simulink library "NLGCToolbox"  (R2017b)
settings: Solver=VariableStepAuto  StartTime=0.0  StopTime=10.0  RelTol=1e-3
undefined symbols (not defined in the file or in its folder): quadModel
libraries: simulink x8, NLGCToolbox x4
settings Model: Creator=hoang  LastModifiedBy=hoang

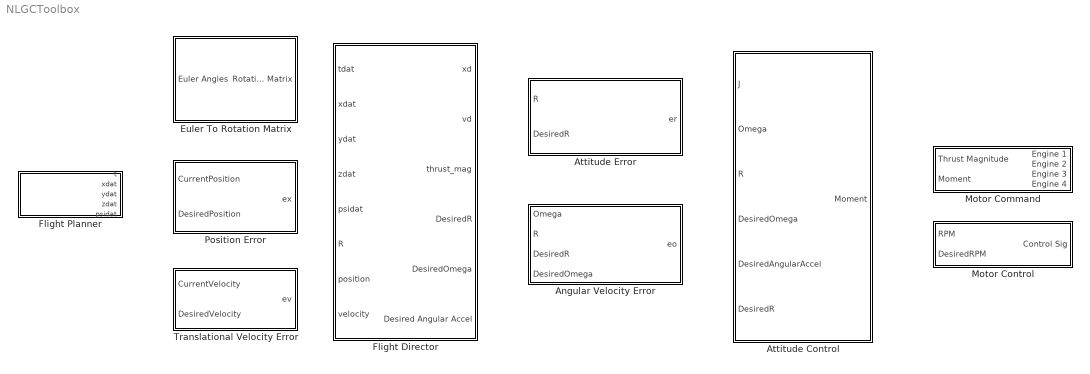
== system NLGCToolbox ==
  Angular Velocity Error : Subsystem
      settings: OpenFcn=set_param(gcbh,'LinkStatus','none');
  Attitude Control : Subsystem  mask{kr=12, ko=4}
      mask prompts: kr "Attitude error gain (Kr)"; ko "Angular velocity error gain (Ko)"
      mask init:
      | set_param(gcb, 'MaskSelfModifiable', 'on');
      settings: OpenFcn=set_param(gcbh,'LinkStatus','none');
  Attitude Error : Subsystem
      settings: OpenFcn=set_param(gcbh,'LinkStatus','none');
  Euler To Rotation Matrix : Subsystem
      settings: OpenFcn=set_param(gcbh,'LinkStatus','none');
  Flight Director : Subsystem  mask{Ts=0, kx=0, kv=0}
      mask prompts: Ts "Sampling Time (Ts)"; kx "Position Control Gain (kx)"; kv "Velocity Control Gain (kv)"
      settings: OpenFcn=set_param(gcbh,'LinkStatus','none');
  "Flight Planner " : Subsystem  mask{t=0, x=0, y=0, z=0, psi=0}
      mask prompts: t "Workspace Time Var"; x "Workspace x Var"; y "Workspace y Var"; z "Workspace z Var"; psi "Workspace psi Var"
      settings: OpenFcn=set_param(gcbh,'LinkStatus','none');
  Motor Command : Subsystem  mask{Ct=0, d=0, Cq=0}
      mask prompts: Ct "Force coefficient (Ct)"; d "Arm's length (d)"; Cq "Reaction torque coefficient (Cq)"
      settings: OpenFcn=set_param(gcbh,'LinkStatus','none');
  Motor Control : Subsystem  mask{k=0, Km=0, Ts=0, T=0, Rdt=0, Rdx=0, b=0}
      mask prompts: k "Velocity Gain (k)"; Km "Motor Amplification (Km)"; Ts "Sampling Time (Ts)"; T "Motor Time Constant (T)"; Rdt "Maximum Output Threshold (Rdt)"; Rdx "Maximum Derivative Threshold (Rdx)"; b "Throttle Bias"
      settings: OpenFcn=set_param(gcbh,'LinkStatus','none');
  Position Error : Subsystem
      settings: OpenFcn=set_param(gcbh,'LinkStatus','none');
  Translational Velocity Error : Subsystem
      settings: OpenFcn=set_param(gcbh,'LinkStatus','none');

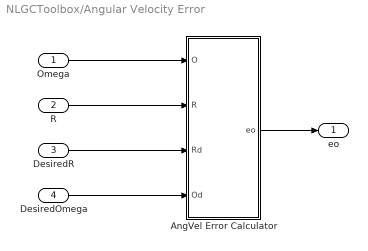
== system NLGCToolbox/Angular Velocity Error ==
  Omega : Inport
  R : Inport  Port=2
  DesiredR : Inport  Port=3
  DesiredOmega : Inport  Port=4
  AngVel Error Calculator : MATLAB Function  TreatAsAtomicUnit=on
  eo : Outport
  wires:
  Omega/1 -> AngVel Error Calculator/1(O)
  R/1 -> AngVel Error Calculator/2(R)
  DesiredR/1 -> AngVel Error Calculator/3(Rd)
  DesiredOmega/1 -> AngVel Error Calculator/4(Od)
  AngVel Error Calculator/1(eo) -> eo/1

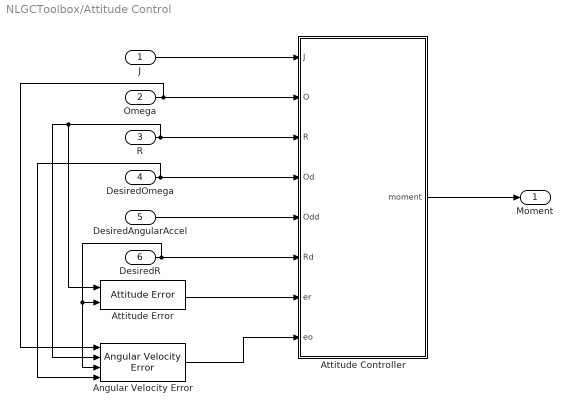
== system NLGCToolbox/Attitude Control ==
  J : Inport
  Omega : Inport  Port=2
  R : Inport  Port=3
  DesiredOmega : Inport  Port=4
  DesiredAngularAccel : Inport  Port=5
  DesiredR : Inport  Port=6
  Angular Velocity Error : NLGCToolbox/Angular Velocity Error
      settings: SourceProductName=Thinh - NLGC for Quadrotor
  Attitude Controller : MATLAB Function  TreatAsAtomicUnit=on
  Attitude Error : NLGCToolbox/Attitude Error
      settings: SourceProductName=Thinh - NLGC for Quadrotor
  Moment : Outport
  wires:
  Attitude Controller/1(moment) -> Moment/1
  DesiredR/1 -> Angular Velocity Error/3, Attitude Error/2, Attitude Controller/6(Rd)
  DesiredAngularAccel/1 -> Attitude Controller/5(Odd)
  DesiredOmega/1 -> Angular Velocity Error/4, Attitude Controller/4(Od)
  R/1 -> Attitude Error/1, Angular Velocity Error/2, Attitude Controller/3(R)
  Omega/1 -> Angular Velocity Error/1, Attitude Controller/2(O)
  J/1 -> Attitude Controller/1(J)
  Attitude Error/1 -> Attitude Controller/7(er)
  Angular Velocity Error/1 -> Attitude Controller/8(eo)

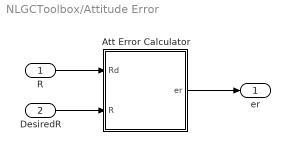
== system NLGCToolbox/Attitude Error ==
  R : Inport
  DesiredR : Inport  Port=2
  Att Error Calculator : MATLAB Function  TreatAsAtomicUnit=on
  er : Outport
  wires:
  Att Error Calculator/1(er) -> er/1
  R/1 -> Att Error Calculator/1(Rd)
  DesiredR/1 -> Att Error Calculator/2(R)

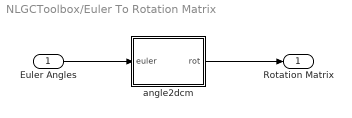
== system NLGCToolbox/Euler To Rotation Matrix ==
  Euler Angles : Inport
  angle2dcm : MATLAB Function  TreatAsAtomicUnit=on
  Rotation Matrix : Outport
  wires:
  Euler Angles/1 -> angle2dcm/1(euler)
  angle2dcm/1(rot) -> Rotation Matrix/1

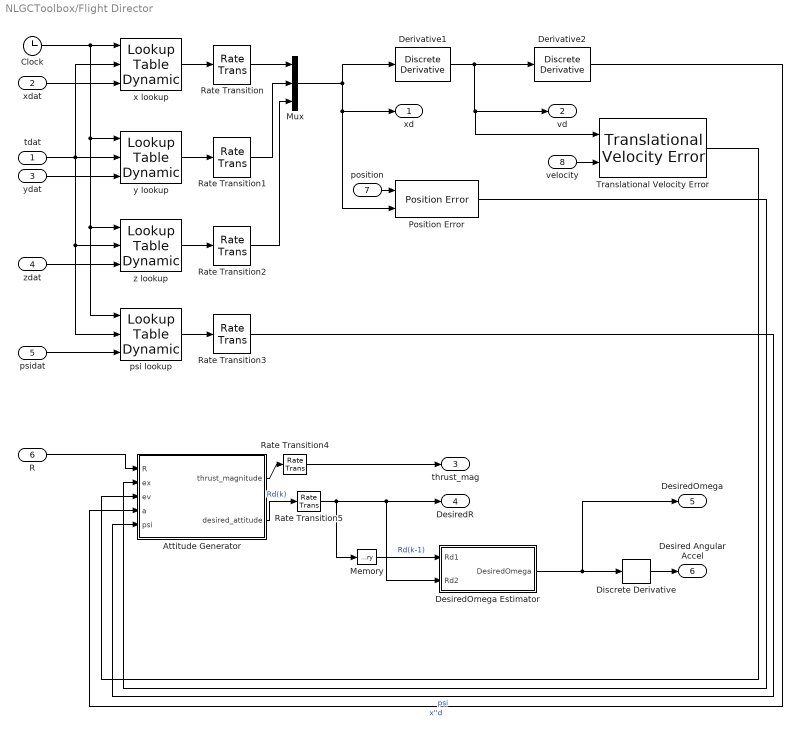
== system NLGCToolbox/Flight Director ==
  tdat : Inport
  xdat : Inport  Port=2
  ydat : Inport  Port=3
  zdat : Inport  Port=4
  psidat : Inport  Port=5
  R : Inport  Port=6
  position : Inport  Port=7
  velocity : Inport  Port=8
  Attitude Generator : MATLAB Function  TreatAsAtomicUnit=on
  Clock : Clock
  Derivative1 : simulink/Discrete/Discrete Derivative  gainval=1.0  ICPrevScaledInput=0.0  OutMin=[]  OutMax=[]  OutDataType=fixdt(1, 16)  OutScaling=2^-10  DoSatur=off
  Derivative2 : simulink/Discrete/Discrete Derivative  gainval=1.0  ICPrevScaledInput=0.0  OutMin=[]  OutMax=[]  OutDataType=fixdt(1, 16)  OutScaling=2^-10  DoSatur=off
  DesiredOmega Estimator : MATLAB Function  TreatAsAtomicUnit=on
  Discrete Derivative : simulink/Discrete/Discrete Derivative  gainval=1.0  ICPrevScaledInput=0.0  OutMin=[]  OutMax=[]  OutDataType=fixdt(1, 16)  OutScaling=2^-10  DoSatur=off
  Memory : Memory
  Mux : Mux  Inputs=3
  Position Error : NLGCToolbox/Position Error
      settings: SourceProductName=Thinh - NLGC for Quadrotor
  Rate Transition{,1..5} (6 alike) : RateTransition  OutPortSampleTime=Ts
  Translational Velocity Error : NLGCToolbox/Translational Velocity Error
      settings: SourceProductName=Thinh - NLGC for Quadrotor
  psi lookup : simulink/Lookup Tables/Lookup Table Dynamic  LookUpMeth=Interpolation-Use End Values  OutDataType=fixdt('double')  OutScaling=[]  OutputDataTypeScalingMode=Specify via dialog  OutDataTypeStr=double  DoSatur=off
      settings: SourceProductName=Simulink
  x lookup : simulink/Lookup Tables/Lookup Table Dynamic  LookUpMeth=Interpolation-Use End Values  OutDataType=fixdt('double')  OutScaling=[]  OutputDataTypeScalingMode=Specify via dialog  OutDataTypeStr=double  DoSatur=off
      settings: SourceProductName=Simulink
  y lookup : simulink/Lookup Tables/Lookup Table Dynamic  LookUpMeth=Interpolation-Use End Values  OutDataType=fixdt('double')  OutScaling=[]  OutputDataTypeScalingMode=Specify via dialog  OutDataTypeStr=double  DoSatur=off
      settings: SourceProductName=Simulink
  z lookup : simulink/Lookup Tables/Lookup Table Dynamic  LookUpMeth=Interpolation-Use End Values  OutDataType=fixdt('double')  OutScaling=[]  OutputDataTypeScalingMode=Specify via dialog  OutDataTypeStr=double  DoSatur=off
      settings: SourceProductName=Simulink
  xd : Outport
  vd : Outport  Port=2
  thrust_mag : Outport  Port=3
  DesiredR : Outport  Port=4
  DesiredOmega : Outport  Port=5
  Desired Angular Accel : Outport  Port=6
  wires:
  tdat/1 -> psi lookup/2, z lookup/2, x lookup/2, y lookup/2
  Clock/1 -> psi lookup/1, z lookup/1, y lookup/1, x lookup/1
  xdat/1 -> x lookup/3
  ydat/1 -> y lookup/3
  zdat/1 -> z lookup/3
  x lookup/1 -> Rate Transition/1
  y lookup/1 -> Rate Transition1/1
  z lookup/1 -> Rate Transition2/1
  Rate Transition/1 -> Mux/1
  Rate Transition1/1 -> Mux/2
  Rate Transition2/1 -> Mux/3
  Derivative1/1 -> Translational Velocity Error/1, vd/1, Derivative2/1
  psi lookup/1 -> Rate Transition3/1
  Derivative2/1 -> Attitude Generator/4(a)  "x''d"
  Rate Transition3/1 -> Attitude Generator/5(psi)  "psi"
  Attitude Generator/1(thrust_magnitude) -> Rate Transition4/1
  Attitude Generator/2(desired_attitude) -> Rate Transition5/1  "Rd(k)"
  R/1 -> Attitude Generator/1(R)
  DesiredOmega Estimator/1(DesiredOmega) -> Discrete Derivative/1, DesiredOmega/1
  Discrete Derivative/1 -> Desired Angular Accel/1
  Rate Transition5/1 -> Memory/1, DesiredOmega Estimator/2(Rd2), DesiredR/1
  Rate Transition4/1 -> thrust_mag/1
  Memory/1 -> DesiredOmega Estimator/1(Rd1)  "Rd(k-1)"
  Mux/1 -> xd/1, Position Error/2, Derivative1/1
  position/1 -> Position Error/1
  Position Error/1 -> Attitude Generator/2(ex)
  velocity/1 -> Translational Velocity Error/2
  Translational Velocity Error/1 -> Attitude Generator/3(ev)
  psidat/1 -> psi lookup/3

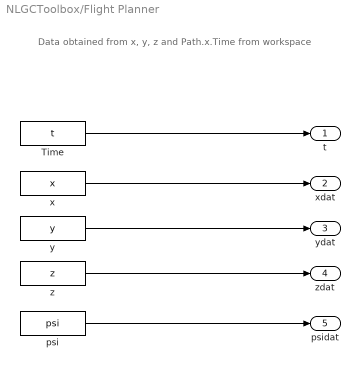
== system NLGCToolbox/Flight Planner  ==
  note: Data obtained from x, y, z and Path.x.Time from workspace
  Time : FromWorkspace  VariableName=t  SampleTime=0
  psi : FromWorkspace  VariableName=psi  SampleTime=0
  x : FromWorkspace  VariableName=x  SampleTime=0
  y : FromWorkspace  VariableName=y  SampleTime=0
  z : FromWorkspace  VariableName=z  SampleTime=0
  t : Outport
  "xdat " : Outport  Port=2
  ydat : Outport  Port=3
  zdat : Outport  Port=4
  psidat : Outport  Port=5
  wires:
  x/1 -> "xdat "/1
  Time/1 -> t/1
  y/1 -> ydat/1
  z/1 -> zdat/1
  psi/1 -> psidat/1

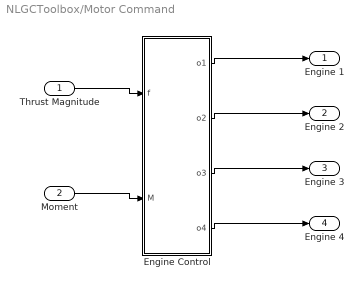
== system NLGCToolbox/Motor Command ==
  " Thrust Magnitude" : Inport
  Moment : Inport  Port=2
  Engine Control : MATLAB Function  TreatAsAtomicUnit=on
  Engine 1 : Outport
  Engine 2 : Outport  Port=2
  Engine 3 : Outport  Port=3
  Engine 4 : Outport  Port=4
  wires:
  " Thrust Magnitude"/1 -> Engine Control/1(f)
  Moment/1 -> Engine Control/2(M)
  Engine Control/1(o1) -> Engine 1/1
  Engine Control/2(o2) -> Engine 2/1
  Engine Control/3(o3) -> Engine 3/1
  Engine Control/4(o4) -> Engine 4/1

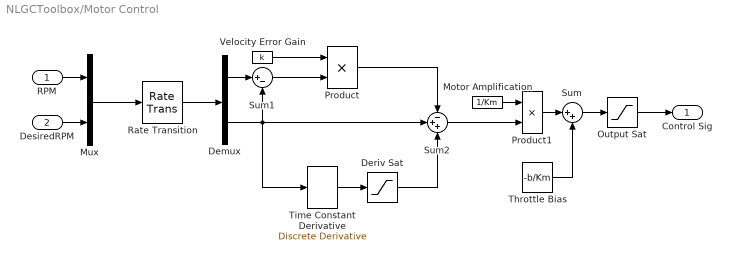
== system NLGCToolbox/Motor Control ==
  RPM : Inport
  DesiredRPM : Inport  Port=2
  Demux : Demux  Outputs=2
  Deriv Sat : Saturate  UpperLimit=Rdx  LowerLimit=-Rdx
  Motor Amplification : Constant  Value=1/Km
  Mux : Mux  Inputs=2
  Output Sat : Saturate  UpperLimit=Rdt  LowerLimit=0
  Product : Product
  Product1 : Product
  Rate Transition : RateTransition  OutPortSampleTime=Ts
  Sum : Sum  Inputs=|++
  Sum1 : Sum  Inputs=|+-
  Sum2 : Sum  Inputs=-++
  Throttle Bias : Constant  Value=-b/Km
  Time Constant Derivative : simulink/Discrete/Discrete Derivative  gainval=T  ICPrevScaledInput=0.0  OutMin=[]  OutMax=[]  OutDataType=fixdt(1, 16)  OutScaling=2^-10  DoSatur=off
  Velocity Error Gain : Constant  Value=k
  Control Sig : Outport
  wires:
  RPM/1 -> Mux/1
  DesiredRPM/1 -> Mux/2
  Mux/1 -> Rate Transition/1
  Rate Transition/1 -> Demux/1
  Demux/2 -> Time Constant Derivative/1, Sum2/2, Sum1/2
  Demux/1 -> Sum1/1
  Sum1/1 -> Product/2
  Velocity Error Gain/1 -> Product/1
  Product/1 -> Sum2/1
  Sum2/1 -> Product1/2
  Motor Amplification/1 -> Product1/1
  Output Sat/1 -> Control Sig/1
  Time Constant Derivative/1 -> Deriv Sat/1
  Deriv Sat/1 -> Sum2/3
  Product1/1 -> Sum/1
  Sum/1 -> Output Sat/1
  Throttle Bias/1 -> Sum/2

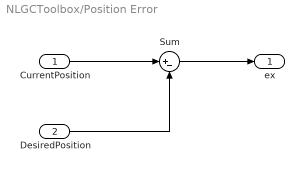
== system NLGCToolbox/Position Error ==
  CurrentPosition : Inport
  DesiredPosition : Inport  Port=2
  Sum : Sum  Inputs=|+-
  ex : Outport
  wires:
  CurrentPosition/1 -> Sum/1
  DesiredPosition/1 -> Sum/2
  Sum/1 -> ex/1

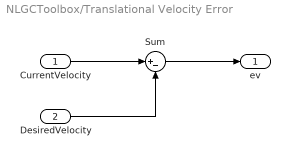
== system NLGCToolbox/Translational Velocity Error ==
  CurrentVelocity : Inport
  DesiredVelocity : Inport  Port=2
  Sum : Sum  Inputs=|+-
  ev : Outport
  wires:
  CurrentVelocity/1 -> Sum/1
  DesiredVelocity/1 -> Sum/2
  Sum/1 -> ev/1

== matlab function NLGCToolbox/Flight Director/Attitude Generator ==
  data: R input size=[3 3]; thrust_magnitude output size=1; ex input size=[3 1]; ev input size=[3 1]; a input size=[3 1]; psi input size=1; desired_attitude output size=[3 3]; kx parameter; kv parameter; quadModel parameter
function [thrust_magnitude,desired_attitude] = fcn(R,ex,ev,a,psi,kx,kv,quadModel)

e3 = [0 0 1]';

desired_thrust = -kx*ex - kv*ev - quadModel.mass*quadModel.g*e3 + quadModel.mass*a;

% Desired Attitude Calculation
z_direction = -desired_thrust/norm(desired_thrust); % b3, from [0 0 1]'
x_direction = findDirection(psi, z_direction, 0); % b1, from [1 0 0]'
y_direction = hat(z_direction)*x_direction; % b2, from [0 1 0]'
desired_attitude = [x_direction y_direction z_direction];
thrust_magnitude = norm(desired_thrust) * (e3'*R'*desired_attitude*e3);

end

% Function to find Promoted Direction Vector
function y = findDirection(psi,thrust_direction,initial_pitch)
Rpsi = angle2dcm(0,initial_pitch,psi,123);
ddv = Rpsi*[1 0 0]'; % Provisional Desired Direction Vector (DDV)
pdv = - (hat(thrust_direction) * (hat(thrust_direction) * ddv)); % Promoted Direction Vector (PDV)
if (isalmost(pdv,zeros(3,1),1e-3))
    Rpsi = angle2dcm(0,initial_pitch,psi,123);
    ddv = Rpsi*[1 0 0]'; % Provisional Desired Direction Vector (DDV)
    pdv = - (hat(thrust_direction) * (hat(thrust_direction) * ddv)); % Promoted Direction Vector (PDV)
    y = pdv/norm(pdv);
else
    y = pdv/norm(pdv);
end
end

== matlab function NLGCToolbox/Attitude Control/Attitude Controller ==
  data: J input size=[3 3]; moment output size=[3 1]; O input size=[3 1]; R input size=[3 3]; Od input size=[3 1]; Odd input size=[3 1]; Rd input size=[3 3]; er input size=[3 1]; eo input size=[3 1]; kr parameter; ko parameter
function moment = fcn(J,O,R,Od,Odd,Rd,er,eo,kr, ko)
moment = hat(O)*(J*O) - J*(hat(O)*R'*Rd*Od - R'*Rd*Odd + kr * er + ko * eo);

== matlab function NLGCToolbox/Euler To Rotation Matrix/angle2dcm ==
  data: euler input size=[3 1]; rot output size=[3 3]
function rot = fcn(euler)
rot = angle2dcm(euler(1), euler(2), euler(3), 123);

== matlab function NLGCToolbox/Angular Velocity Error/AngVel Error Calculator ==
  data: O input size=[3 1]; eo output size=[3 1]; R input size=[3 3]; Rd input size=[3 3]; Od input size=[3 1]
function eo = fcn(O, R, Rd, Od)
eo = O-R'*Rd*Od;

== matlab function NLGCToolbox/Attitude Error/Att Error Calculator ==
  data: er output size=[3 1]; Rd input size=[3 3]; R input size=[3 3]
function er  = fcn(Rd, R)
er = 1/2*vee(Rd'*R-R'*Rd);

== matlab function NLGCToolbox/Flight Director/DesiredOmega Estimator ==
  data: Rd1 input size=[3 3]; DesiredOmega output size=[3 1]; Rd2 input size=[3 3]
function DesiredOmega = fcn(Rd1,Rd2)
Rd_delta = Rd2*Rd1';
DesiredOmega = vee(Rd_delta);

== matlab function NLGCToolbox/Motor Command/Engine Control ==
  data: f input size=1; o1 output size=1; M input size=[3 1]; o2 output size=1; o3 output size=1; o4 output size=1; Ct parameter; d parameter; Cq parameter
function [o1,o2,o3,o4] = fcn(f,M,Ct, d, Cq)
force = [f; M];
gamma = [Ct Ct Ct Ct;
    0 d*Ct 0 -d*Ct;
    -d*Ct 0 d*Ct 0;
    -Cq Cq -Cq Cq];
omega = sqrt(force\gamma);
o1=omega(1);
o2=omega(2);
o3=omega(3);
o4=omega(4);
